simulink model "pendolofortests"  (R2018b)
settings: Solver=VariableStepAuto  StartTime=0.0  StopTime=35  MaxStep=0.2  RelTol=1e-10
values from neighbouring files (symbols this model uses):
  g = 9.81    [main.m]
  Jm = 3.1e-7    (= 3.1e-07)    [main.m]
  Jp = 1774.274e-6    (= 0.001774274)    [main.m]
  Kf = 7.44e-3    (= 0.00744)    [main.m]
  La = 35e-6    (= 3.5e-05)    [main.m]
  lb = 141.451e-3    (= 0.141451)    [main.m]
  m = 135.4e-3    (= 0.1354)    [main.m]
  M = 879.5e-3    (= 0.8795)    [main.m]
  Ra = 3.92    [main.m]
  Rg = (13.55+11.04)/4    (= 6.1475)    [main.m]
  rt = 0.01    [main.m]
undefined symbols (not defined in the file or in its folder): p1, p2
settings Model: Creator=lelli  LastModifiedBy=Giorgio
settings SFSimCC: SimUseLocalCustomCode=off
settings RTWCC: RTWUseLocalCustomCode=off

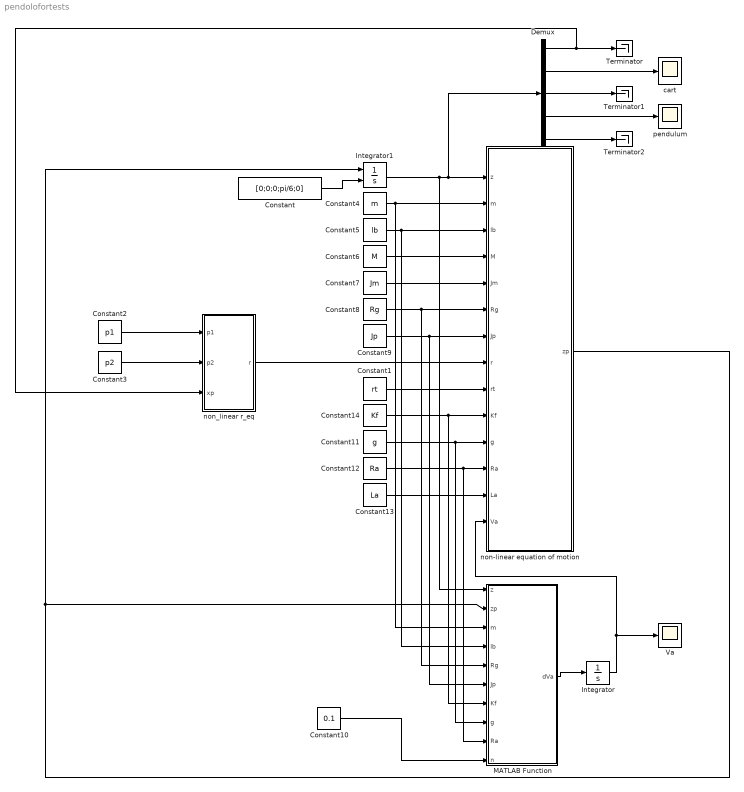
== system pendolofortests ==
  Constant : Constant  Value=[0;0;0;pi/6;0]
  Constant1 : Constant  Value=rt
  Constant10 : Constant  Value=0.1
  Constant11 : Constant  Value=g
  Constant12 : Constant  Value=Ra
  Constant13 : Constant  Value=La
  Constant14 : Constant  Value=Kf
  Constant2 : Constant  Value=p1
  Constant3 : Constant  Value=p2
  Constant4 : Constant  Value=m
  Constant5 : Constant  Value=lb
  Constant6 : Constant  Value=M
  Constant7 : Constant  Value=Jm
  Constant8 : Constant  Value=Rg
  Constant9 : Constant  Value=Jp
  Demux : Demux  Outputs=5
  Integrator : Integrator
  Integrator1 : Integrator  InitialConditionSource=external
  MATLAB Function : MATLAB Function  TreatAsAtomicUnit=on
  Terminator : Terminator
  Terminator1 : Terminator
  Terminator2 : Terminator
  "Va " : Scope
  cart : Scope
  "non-linear equation of motion " : MATLAB Function  TreatAsAtomicUnit=on
  "non_linear r_eq " : MATLAB Function  TreatAsAtomicUnit=on
  pendulum : Scope
  wires:
  Constant4/1 -> MATLAB Function/3(m), "non-linear equation of motion "/2(m)
  Constant5/1 -> MATLAB Function/4(lb), "non-linear equation of motion "/3(lb)
  Constant6/1 -> "non-linear equation of motion "/4(M)
  Constant7/1 -> "non-linear equation of motion "/5(Jm)
  Constant8/1 -> MATLAB Function/5(Rg), "non-linear equation of motion "/6(Rg)
  Constant9/1 -> MATLAB Function/6(Jp), "non-linear equation of motion "/7(Jp)
  Constant14/1 -> MATLAB Function/7(Kf), "non-linear equation of motion "/10(Kf)
  Constant11/1 -> MATLAB Function/8(g), "non-linear equation of motion "/11(g)
  Constant12/1 -> MATLAB Function/9(Ra), "non-linear equation of motion "/12(Ra)
  Constant13/1 -> "non-linear equation of motion "/13(La)
  Demux/2 -> cart/1
  Constant1/1 -> "non-linear equation of motion "/9(rt)
  "non_linear r_eq "/1(r) -> "non-linear equation of motion "/8(r)
  Constant2/1 -> "non_linear r_eq "/1(p1)
  Constant3/1 -> "non_linear r_eq "/2(p2)
  Constant/1 -> Integrator1/2
  Integrator1/1 -> MATLAB Function/1(z), Demux/1, "non-linear equation of motion "/1(z)
  "non-linear equation of motion "/1(zp) -> Integrator1/1, MATLAB Function/2(zp)
  Demux/4 -> pendulum/1
  Demux/3 -> Terminator1/1
  Demux/5 -> Terminator2/1
  Demux/1 -> "non_linear r_eq "/3(xp), Terminator/1
  Constant10/1 -> MATLAB Function/10(n)
  Integrator/1 -> "non-linear equation of motion "/14(Va), "Va "/1
  MATLAB Function/1(dVa) -> Integrator/1

== matlab function pendolofortests/non_linear r_eq  ==
  data: p1 input; r output; p2 input; xp input
function r  = r_eq(p1,p2,xp)
%non linear relationship between velocity and cart dumping
%p1 is the slope of linear approximation of force measured
%p2 is the intercept of linear approximation of force measured
%xp is the instantaneous velocity 
if xp>1e-16 || xp<-1e-16
    r=2*p2/pi*atan(100*xp)/xp + p1;
else
    r=2*p2/pi*100+p1;
end
end

== matlab function pendolofortests/non-linear equation of motion  ==
  data: z input; m input; zp output; lb input; M input; Jm input; Rg input; Jp input; r input; rt input; Kf input; g input; Ra input; La input; Va input
function zp = pendulum(z,m,lb,M,Jm,Rg,Jp,r,rt,Kf,g,Ra,La,Va)
xp=z(1);
tetap=z(3);
teta=z(4);
Ia=z(5);

A=[(M + m + Jm/Rg^2) 0 m*cos(teta)*lb 0 0; 
   0 1 0 0 0; 
   m*cos(teta)*lb 0 (Jp + m*lb^2) 0 0; 
   0 0 0 1 0; 
   0 0 0 0 La];

zp =(A)\[m*sin(teta)*lb*tetap^2 - r*xp + Kf*Ia/Rg;
         xp;
         - lb*m*g*sin(teta) - rt*tetap;
         tetap;
         Va - Ra*Ia - Kf/Rg*xp];
end

== matlab function pendolofortests/MATLAB Function ==
  data: z input; zp input; dVa output; m input; lb input; Rg input; Jp input; Kf input; g input; Ra input; n input
function dVa = swup(z,zp,m,lb,Rg,Jp,Kf,g,Ra,n)
E0=m*g*lb;
thp=z(3);
th=z(4);
Iap=zp(5);
E=(1/2)*(Jp+m*lb^2)*thp^2+m*g*lb*(cos(th)-1);
% n is a sort of gain for swing up speed
dVa=n*(Kf/Rg)*g*sign((E-E0)*thp*cos(th))+Ra*Iap;
end
